simulink model "afsMatrixBeam"  (R2019b)
settings: Solver=FixedStepDiscrete  StartTime=0.0  StopTime=inf  RelTol=1e-3  EnableMultiTasking=on
libraries: SCANeR_API x3
settings Model: Creator=davendano  LastModifiedBy=lpfeffer
settings DataIOCC: LimitDataPoints=on  SaveFormat=Array  ReturnWorkspaceOutputs=off
settings OptimizationCC: LifeSpan=inf
settings DebuggingCC: UnderspecifiedInitializationDetection=Classic  MergeDetectMultiDrivingBlocksExec=none  SolverPrmCheckMsg=warning  SFUnexpectedBacktrackingDiag=warning  SFNoUnconditionalDefaultTransitionDiag=warning  SFExecutionAtInitializationDiag=none  ArithmeticOperatorsInVariantConditions=warning
settings HardwareCC: ProdBitPerPointer=32  ProdBitPerSizeT=32  ProdBitPerPtrDiffT=32  ProdLargestAtomicFloat=None  ProdIntDivRoundTo=Undefined  ProdEndianess=Unspecified  ProdWordSize=32  ProdHWDeviceType=32-bit Generic
settings ModelReferenceCC: PropagateSignalLabelsOutOfModel=off
settings SFSimCC: SimUseLocalCustomCode=off  CustomCodeUndefinedFunction=UseInterfaceOnly
settings RTWCC: Description=OKTAL AFS SCANeR Real-Time Target  SystemTargetFile=grt_CallasPlugin.tlc  TemplateMakefile=grt_moduleOktal  RTWUseLocalCustomCode=off
settings CodeAppCC: StateflowObjectComments=on
settings STFCustomTargetCC: ModelReferenceCompliant=off  GeneratePreprocessorConditionals=Disable all  CombineOutputUpdateFcns=on  MatFileLogging=on  CPPClassGenCompliant=on  SystemTargetFile=grt_CallasPlugin.tlc
settings GRTTargetCC: TargetLangStandard=C89/C90 (ANSI)  ModelReferenceCompliant=off  ParMdlRefBuildCompliant=off  CompOptLevelCompliant=off  ConcurrentExecutionCompliant=off  GeneratePreprocessorConditionals=Disable all  UseToolchainInfoCompliant=off
settings ConfigComp: CovMetricSettings=dw  CovHtmlReporting=on  CovSaveCumulativeToWorkspaceVar=on  CovSaveSingleToWorkspaceVar=on  CovExternalEMLEnable=off

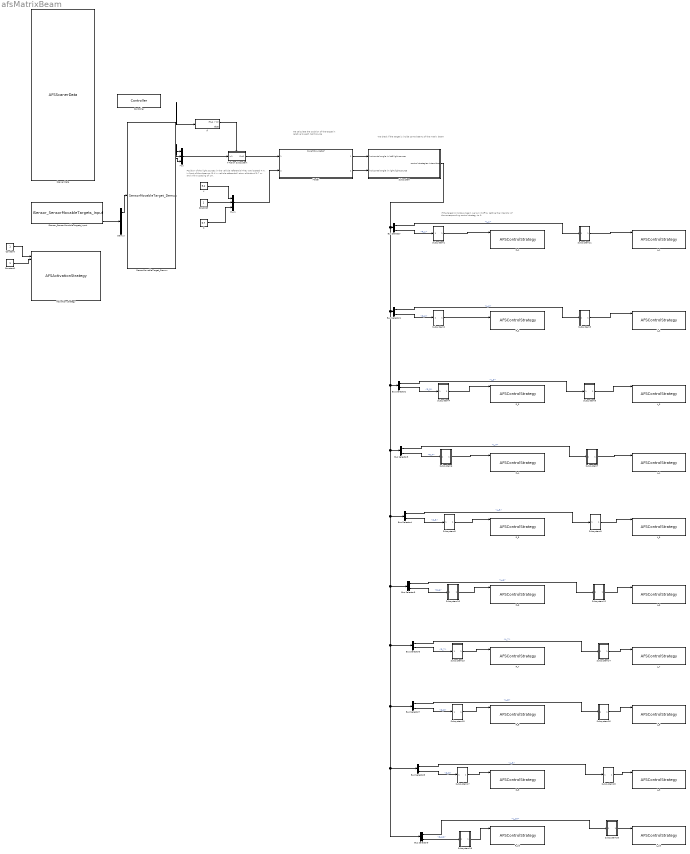
== system afsMatrixBeam ==
  note: If the target is inside a beam we turn it off
      | by setting the intensity of the corresponding control strategy to 0.
  note: We check if the target is inside some beams of the matrix beam
  note: We calculate the position of the target in
      | relative to each light source
  note: Position of the light sources in the vehicle referential
      | They are located 4 m. in front of the observer (5.4 in vehicle referential)
      | at an altitude of 0.7 m. and with a spacing of 1m.
  Activation strategy : S-Function  InitFcn=try, set_param(gcb,'FunctionName','AFSActivationStrategy'), end  FunctionName=AFSActivationStrategy  SFunctionDeploymentMode=off  EnableBusSupport=off  mask(S-Function Builder){}
      mask init:
      | val = [[.9  0.75 0.75 1 1 .9 .9 1]',[1 1 0.75 0.75 .9 .9 1 .9]'];try , sys = get_param(gcb,'SfunBuilderFcnName');if isempty(sys), sys = get_param(gcb,'FunctionName'); end,catch, sys = get_param(gcb,'FunctionName'); end
      settings: CopyFcn=set_param(gcbh,'LinkStatus','none')  PreSaveFcn=try, set_param(gcb,'FunctionName','AFSActivationStrategy'), end
      mask Display:
      | port_label('input',1,'LowBeam')
      | port_label('input',2,'HighBeam')
      | port_label('input',3,'MotorWay')
      | port_label('input',4,'Town')
      | port_label('input',5,'Traffic')
      | port_label('input',6,'AdverseWeather')
      | port_label('input',7,'TurnIndicator')
      | port_label('input',8,'DayTimeRunningLight')
      | port_label('input',9,'ProgressiveBendingLight')
      | port_label('input',10,'CustomBeam1')
      | port_label('input',11,'CustomBeam2')
      | port_label('input',12,'CustomBeam3')
      | fprintf('ACTIVATION\n STRATEGY\n')
  Bus Selector : BusSelector  OutputSignals=L.L_1,R.R_1
  Bus Selector1 : BusSelector  OutputSignals=L.L_2,R.R_2
  Bus Selector2 : BusSelector  OutputSignals=L.L_3,R.R_3
  Bus Selector3 : BusSelector  OutputSignals=L.L_4,R.R_4
  Bus Selector4 : BusSelector  OutputSignals=L.L_5,R.R_5
  Bus Selector5 : BusSelector  OutputSignals=L.L_6,R.R_6
  Bus Selector6 : BusSelector  OutputSignals=L.L_7,R.R_7
  Bus Selector7 : BusSelector  OutputSignals=L.L_8,R.R_8
  Bus Selector8 : BusSelector  OutputSignals=L.L_9,R.R_9
  Bus Selector9 : BusSelector  OutputSignals=L.L_10,R.R_10
  Constant : Constant
  Constant1 : Constant
  Controller : SCANeR_API/Controller  Priority=1  Config='SAMPLE_2022_HEADLIGHTS'  ProcName='SIMULINK'  Frequency=100  NetworkOutputFrequency=10  TimeOut=30  IsSynchronized=off
      settings: SourceProductName=SCANeR API
  Demux : Demux  Outputs=[41 41 41 10373]
  ISensor_SensorMovableTargets_Input : SCANeR_API/Network inputs/ISensor/ISensor_SensorMovableTargets_Input  Priority=2  ev=off  globalId=100000
      settings: SourceProductName=SCANeR API
  If : If
  If Action Subsystem : Subsystem  TreatAsAtomicUnit=on
  L_1 : S-Function  InitFcn=try, set_param(gcb,'FunctionName','AFSControlStrategy'), end  FunctionName=AFSControlStrategy  SFunctionDeploymentMode=off  EnableBusSupport=off  mask(S-Function Builder){}
      mask init: same as afsMatrixBeam/Activation strategy
      settings: CopyFcn=set_param(gcbh,'LinkStatus','none')  PreSaveFcn=try, set_param(gcb,'FunctionName','AFSControlStrategy'), end
      mask Display:
      | port_label('input',1,'Intensity')
      | port_label('input',2,'Heading')
      | port_label('input',3,'Pitch')
      | port_label('input',4,'Roll')
      | fprintf('CONTROL\n STRATEGY\n name:%s\n',get_param(gcb, 'Name'))
  L_10 : S-Function  InitFcn=try, set_param(gcb,'FunctionName','AFSControlStrategy'), end  FunctionName=AFSControlStrategy  SFunctionDeploymentMode=off  EnableBusSupport=off  mask(S-Function Builder){}
      mask init: same as afsMatrixBeam/Activation strategy
      settings: CopyFcn=set_param(gcbh,'LinkStatus','none')  PreSaveFcn=try, set_param(gcb,'FunctionName','AFSControlStrategy'), end
      mask Display:
      | port_label('input',1,'Intensity')
      | port_label('input',2,'Heading')
      | port_label('input',3,'Pitch')
      | port_label('input',4,'Roll')
      | fprintf('CONTROL\n STRATEGY\n name:%s\n',get_param(gcb, 'Name'))
  L_2 : S-Function  InitFcn=try, set_param(gcb,'FunctionName','AFSControlStrategy'), end  FunctionName=AFSControlStrategy  SFunctionDeploymentMode=off  EnableBusSupport=off  mask(S-Function Builder){}
      mask init: same as afsMatrixBeam/Activation strategy
      settings: CopyFcn=set_param(gcbh,'LinkStatus','none')  PreSaveFcn=try, set_param(gcb,'FunctionName','AFSControlStrategy'), end
      mask Display:
      | port_label('input',1,'Intensity')
      | port_label('input',2,'Heading')
      | port_label('input',3,'Pitch')
      | port_label('input',4,'Roll')
      | fprintf('CONTROL\n STRATEGY\n name:%s\n',get_param(gcb, 'Name'))
  L_3 : S-Function  InitFcn=try, set_param(gcb,'FunctionName','AFSControlStrategy'), end  FunctionName=AFSControlStrategy  SFunctionDeploymentMode=off  EnableBusSupport=off  mask(S-Function Builder){}
      mask init: same as afsMatrixBeam/Activation strategy
      settings: CopyFcn=set_param(gcbh,'LinkStatus','none')  PreSaveFcn=try, set_param(gcb,'FunctionName','AFSControlStrategy'), end
      mask Display:
      | port_label('input',1,'Intensity')
      | port_label('input',2,'Heading')
      | port_label('input',3,'Pitch')
      | port_label('input',4,'Roll')
      | fprintf('CONTROL\n STRATEGY\n name:%s\n',get_param(gcb, 'Name'))
  L_4 : S-Function  InitFcn=try, set_param(gcb,'FunctionName','AFSControlStrategy'), end  FunctionName=AFSControlStrategy  SFunctionDeploymentMode=off  EnableBusSupport=off  mask(S-Function Builder){}
      mask init: same as afsMatrixBeam/Activation strategy
      settings: CopyFcn=set_param(gcbh,'LinkStatus','none')  PreSaveFcn=try, set_param(gcb,'FunctionName','AFSControlStrategy'), end
      mask Display:
      | port_label('input',1,'Intensity')
      | port_label('input',2,'Heading')
      | port_label('input',3,'Pitch')
      | port_label('input',4,'Roll')
      | fprintf('CONTROL\n STRATEGY\n name:%s\n',get_param(gcb, 'Name'))
  L_5 : S-Function  InitFcn=try, set_param(gcb,'FunctionName','AFSControlStrategy'), end  FunctionName=AFSControlStrategy  SFunctionDeploymentMode=off  EnableBusSupport=off  mask(S-Function Builder){}
      mask init: same as afsMatrixBeam/Activation strategy
      settings: CopyFcn=set_param(gcbh,'LinkStatus','none')  PreSaveFcn=try, set_param(gcb,'FunctionName','AFSControlStrategy'), end
      mask Display:
      | port_label('input',1,'Intensity')
      | port_label('input',2,'Heading')
      | port_label('input',3,'Pitch')
      | port_label('input',4,'Roll')
      | fprintf('CONTROL\n STRATEGY\n name:%s\n',get_param(gcb, 'Name'))
  L_6 : S-Function  InitFcn=try, set_param(gcb,'FunctionName','AFSControlStrategy'), end  FunctionName=AFSControlStrategy  SFunctionDeploymentMode=off  EnableBusSupport=off  mask(S-Function Builder){}
      mask init: same as afsMatrixBeam/Activation strategy
      settings: CopyFcn=set_param(gcbh,'LinkStatus','none')  PreSaveFcn=try, set_param(gcb,'FunctionName','AFSControlStrategy'), end
      mask Display:
      | port_label('input',1,'Intensity')
      | port_label('input',2,'Heading')
      | port_label('input',3,'Pitch')
      | port_label('input',4,'Roll')
      | fprintf('CONTROL\n STRATEGY\n name:%s\n',get_param(gcb, 'Name'))
  L_7 : S-Function  InitFcn=try, set_param(gcb,'FunctionName','AFSControlStrategy'), end  FunctionName=AFSControlStrategy  SFunctionDeploymentMode=off  EnableBusSupport=off  mask(S-Function Builder){}
      mask init: same as afsMatrixBeam/Activation strategy
      settings: CopyFcn=set_param(gcbh,'LinkStatus','none')  PreSaveFcn=try, set_param(gcb,'FunctionName','AFSControlStrategy'), end
      mask Display:
      | port_label('input',1,'Intensity')
      | port_label('input',2,'Heading')
      | port_label('input',3,'Pitch')
      | port_label('input',4,'Roll')
      | fprintf('CONTROL\n STRATEGY\n name:%s\n',get_param(gcb, 'Name'))
  L_8 : S-Function  InitFcn=try, set_param(gcb,'FunctionName','AFSControlStrategy'), end  FunctionName=AFSControlStrategy  SFunctionDeploymentMode=off  EnableBusSupport=off  mask(S-Function Builder){}
      mask init: same as afsMatrixBeam/Activation strategy
      settings: CopyFcn=set_param(gcbh,'LinkStatus','none')  PreSaveFcn=try, set_param(gcb,'FunctionName','AFSControlStrategy'), end
      mask Display:
      | port_label('input',1,'Intensity')
      | port_label('input',2,'Heading')
      | port_label('input',3,'Pitch')
      | port_label('input',4,'Roll')
      | fprintf('CONTROL\n STRATEGY\n name:%s\n',get_param(gcb, 'Name'))
  L_9 : S-Function  InitFcn=try, set_param(gcb,'FunctionName','AFSControlStrategy'), end  FunctionName=AFSControlStrategy  SFunctionDeploymentMode=off  EnableBusSupport=off  mask(S-Function Builder){}
      mask init: same as afsMatrixBeam/Activation strategy
      settings: CopyFcn=set_param(gcbh,'LinkStatus','none')  PreSaveFcn=try, set_param(gcb,'FunctionName','AFSControlStrategy'), end
      mask Display:
      | port_label('input',1,'Intensity')
      | port_label('input',2,'Heading')
      | port_label('input',3,'Pitch')
      | port_label('input',4,'Roll')
      | fprintf('CONTROL\n STRATEGY\n name:%s\n',get_param(gcb, 'Name'))
  Model : ModelReference  ModelNameDialog=toLightSourceRef.slx  SimulationMode=Normal  ModelReferenceVersion=1.14
  Mux : Mux  Inputs=3
  Mux1 : Mux  Inputs=3
  R_1 : S-Function  InitFcn=try, set_param(gcb,'FunctionName','AFSControlStrategy'), end  FunctionName=AFSControlStrategy  SFunctionDeploymentMode=off  EnableBusSupport=off  mask(S-Function Builder){}
      mask init: same as afsMatrixBeam/Activation strategy
      settings: CopyFcn=set_param(gcbh,'LinkStatus','none')  PreSaveFcn=try, set_param(gcb,'FunctionName','AFSControlStrategy'), end
      mask Display:
      | port_label('input',1,'Intensity')
      | port_label('input',2,'Heading')
      | port_label('input',3,'Pitch')
      | port_label('input',4,'Roll')
      | fprintf('CONTROL\n STRATEGY\n name:%s\n',get_param(gcb, 'Name'))
  R_10 : S-Function  InitFcn=try, set_param(gcb,'FunctionName','AFSControlStrategy'), end  FunctionName=AFSControlStrategy  SFunctionDeploymentMode=off  EnableBusSupport=off  mask(S-Function Builder){}
      mask init: same as afsMatrixBeam/Activation strategy
      settings: CopyFcn=set_param(gcbh,'LinkStatus','none')  PreSaveFcn=try, set_param(gcb,'FunctionName','AFSControlStrategy'), end
      mask Display:
      | port_label('input',1,'Intensity')
      | port_label('input',2,'Heading')
      | port_label('input',3,'Pitch')
      | port_label('input',4,'Roll')
      | fprintf('CONTROL\n STRATEGY\n name:%s\n',get_param(gcb, 'Name'))
  R_2 : S-Function  InitFcn=try, set_param(gcb,'FunctionName','AFSControlStrategy'), end  FunctionName=AFSControlStrategy  SFunctionDeploymentMode=off  EnableBusSupport=off  mask(S-Function Builder){}
      mask init: same as afsMatrixBeam/Activation strategy
      settings: CopyFcn=set_param(gcbh,'LinkStatus','none')  PreSaveFcn=try, set_param(gcb,'FunctionName','AFSControlStrategy'), end
      mask Display:
      | port_label('input',1,'Intensity')
      | port_label('input',2,'Heading')
      | port_label('input',3,'Pitch')
      | port_label('input',4,'Roll')
      | fprintf('CONTROL\n STRATEGY\n name:%s\n',get_param(gcb, 'Name'))
  R_3 : S-Function  InitFcn=try, set_param(gcb,'FunctionName','AFSControlStrategy'), end  FunctionName=AFSControlStrategy  SFunctionDeploymentMode=off  EnableBusSupport=off  mask(S-Function Builder){}
      mask init: same as afsMatrixBeam/Activation strategy
      settings: CopyFcn=set_param(gcbh,'LinkStatus','none')  PreSaveFcn=try, set_param(gcb,'FunctionName','AFSControlStrategy'), end
      mask Display:
      | port_label('input',1,'Intensity')
      | port_label('input',2,'Heading')
      | port_label('input',3,'Pitch')
      | port_label('input',4,'Roll')
      | fprintf('CONTROL\n STRATEGY\n name:%s\n',get_param(gcb, 'Name'))
  R_4 : S-Function  InitFcn=try, set_param(gcb,'FunctionName','AFSControlStrategy'), end  FunctionName=AFSControlStrategy  SFunctionDeploymentMode=off  EnableBusSupport=off  mask(S-Function Builder){}
      mask init: same as afsMatrixBeam/Activation strategy
      settings: CopyFcn=set_param(gcbh,'LinkStatus','none')  PreSaveFcn=try, set_param(gcb,'FunctionName','AFSControlStrategy'), end
      mask Display:
      | port_label('input',1,'Intensity')
      | port_label('input',2,'Heading')
      | port_label('input',3,'Pitch')
      | port_label('input',4,'Roll')
      | fprintf('CONTROL\n STRATEGY\n name:%s\n',get_param(gcb, 'Name'))
  R_5 : S-Function  InitFcn=try, set_param(gcb,'FunctionName','AFSControlStrategy'), end  FunctionName=AFSControlStrategy  SFunctionDeploymentMode=off  EnableBusSupport=off  mask(S-Function Builder){}
      mask init: same as afsMatrixBeam/Activation strategy
      settings: CopyFcn=set_param(gcbh,'LinkStatus','none')  PreSaveFcn=try, set_param(gcb,'FunctionName','AFSControlStrategy'), end
      mask Display:
      | port_label('input',1,'Intensity')
      | port_label('input',2,'Heading')
      | port_label('input',3,'Pitch')
      | port_label('input',4,'Roll')
      | fprintf('CONTROL\n STRATEGY\n name:%s\n',get_param(gcb, 'Name'))
  R_6 : S-Function  InitFcn=try, set_param(gcb,'FunctionName','AFSControlStrategy'), end  FunctionName=AFSControlStrategy  SFunctionDeploymentMode=off  EnableBusSupport=off  mask(S-Function Builder){}
      mask init: same as afsMatrixBeam/Activation strategy
      settings: CopyFcn=set_param(gcbh,'LinkStatus','none')  PreSaveFcn=try, set_param(gcb,'FunctionName','AFSControlStrategy'), end
      mask Display:
      | port_label('input',1,'Intensity')
      | port_label('input',2,'Heading')
      | port_label('input',3,'Pitch')
      | port_label('input',4,'Roll')
      | fprintf('CONTROL\n STRATEGY\n name:%s\n',get_param(gcb, 'Name'))
  R_7 : S-Function  InitFcn=try, set_param(gcb,'FunctionName','AFSControlStrategy'), end  FunctionName=AFSControlStrategy  SFunctionDeploymentMode=off  EnableBusSupport=off  mask(S-Function Builder){}
      mask init: same as afsMatrixBeam/Activation strategy
      settings: CopyFcn=set_param(gcbh,'LinkStatus','none')  PreSaveFcn=try, set_param(gcb,'FunctionName','AFSControlStrategy'), end
      mask Display:
      | port_label('input',1,'Intensity')
      | port_label('input',2,'Heading')
      | port_label('input',3,'Pitch')
      | port_label('input',4,'Roll')
      | fprintf('CONTROL\n STRATEGY\n name:%s\n',get_param(gcb, 'Name'))
  R_8 : S-Function  InitFcn=try, set_param(gcb,'FunctionName','AFSControlStrategy'), end  FunctionName=AFSControlStrategy  SFunctionDeploymentMode=off  EnableBusSupport=off  mask(S-Function Builder){}
      mask init: same as afsMatrixBeam/Activation strategy
      settings: CopyFcn=set_param(gcbh,'LinkStatus','none')  PreSaveFcn=try, set_param(gcb,'FunctionName','AFSControlStrategy'), end
      mask Display:
      | port_label('input',1,'Intensity')
      | port_label('input',2,'Heading')
      | port_label('input',3,'Pitch')
      | port_label('input',4,'Roll')
      | fprintf('CONTROL\n STRATEGY\n name:%s\n',get_param(gcb, 'Name'))
  R_9 : S-Function  InitFcn=try, set_param(gcb,'FunctionName','AFSControlStrategy'), end  FunctionName=AFSControlStrategy  SFunctionDeploymentMode=off  EnableBusSupport=off  mask(S-Function Builder){}
      mask init: same as afsMatrixBeam/Activation strategy
      settings: CopyFcn=set_param(gcbh,'LinkStatus','none')  PreSaveFcn=try, set_param(gcb,'FunctionName','AFSControlStrategy'), end
      mask Display:
      | port_label('input',1,'Intensity')
      | port_label('input',2,'Heading')
      | port_label('input',3,'Pitch')
      | port_label('input',4,'Roll')
      | fprintf('CONTROL\n STRATEGY\n name:%s\n',get_param(gcb, 'Name'))
  SPACING : Constant
  Scaner Data : S-Function  InitFcn=try, set_param(gcb,'FunctionName','AFSScanerData'), end  FunctionName=AFSScanerData  Parameters=Frequency  SFunctionDeploymentMode=off  EnableBusSupport=off  mask(S-Function Builder){Frequency=100}
      mask prompts: Frequency "Frequency (Hz) (use 0 when used with SCANeR API)"
      mask init: same as afsMatrixBeam/Activation strategy
      settings: CopyFcn=set_param(gcbh,'LinkStatus','none')  PreSaveFcn=try, set_param(gcb,'FunctionName','AFSScanerData'), end
      mask Display:
      | port_label('output',1,'Speed')
      | port_label('output',2,'SteeringWheelAngle')
      | port_label('output',3,'CurrentCurveCurvature')
      | port_label('output',4,'CurveCurvatureAtXMeters')
      | port_label('output',5,'TheoreticalTime')
      | port_label('output',6,'MeasuredTime')
      | port_label('output',7,'X')
      | port_label('output',8,'Y')
      | port_label('output',9,'Z')
      | port_label('output',10,'Heading')
      | port_label('output',11,'Pitch')
      | port_label('output',12,'Roll')
      | port_label('output',13,'HeadingRelativeToTheRoad')
      | port_label('output',14,'GeographicClassification')
      | port_label('output',15,'GearBox')
      | port_label('output',16,'Indicators')
      | port_label('output',17,'Warning')
      | port_label('output',18,'LightStatus')
      | port_label('output',19,'LongitudinalAcceleration')
      | port_label('output',20,'DistanceToNextVehicleInSameDirection')
      | port_label('output',21,'DistanceToNextVehicleInOppositeDirection')
      | port_label('output',22,'SnowLevel')
      | port_label('output',23,'RainLevel')
      | port_label('output',24,'FogDistance')
      | port_label('output',25,'BrakePedal')
      | port_label('output',26,'AcceleratorPedal')
      | port_label('output',27,'VehicleLoad')
      | port_label('output',28,'RemoteHeightAdjustmentHeadlamp')
      | port_label('output',29,'SteerAngle')
      | port_label('output',30,'Wheelbase')
      | port_label('output',31,'AngularVelocityHeading')
      | port_label('output',32,'Traffic')
      | port_label('output',33,'CustomInput')
      | port_label('output',34,'CustomOutput')
      | fprintf('SCANeR\n DATA\n')
  SensorMovableTarget_Demux : SCANeR_API/Structures/SensorMovableTarget_Demux
      settings: SourceProductName=SCANeR API
  Subsystem : Subsystem
  Subsystem1 : Subsystem
  Subsystem10 : Subsystem
  Subsystem11 : Subsystem
  Subsystem12 : Subsystem
  Subsystem13 : Subsystem
  Subsystem14 : Subsystem
  Subsystem15 : Subsystem
  Subsystem16 : Subsystem
  Subsystem17 : Subsystem
  Subsystem18 : Subsystem
  Subsystem19 : Subsystem
  Subsystem2 : Subsystem
  Subsystem20 : Subsystem
  Subsystem3 : Subsystem
  Subsystem4 : Subsystem
  Subsystem5 : Subsystem
  Subsystem6 : Subsystem
  Subsystem7 : Subsystem
  Subsystem8 : Subsystem
  Subsystem9 : Subsystem
  X : Constant  Value=5.4
  Z : Constant  Value=0.7
  wires:
  Constant/1 -> Activation strategy/1
  Constant1/1 -> Activation strategy/2
  ISensor_SensorMovableTargets_Input/6 -> Demux/1
  Demux/1 -> SensorMovableTarget_Demux/1
  SensorMovableTarget_Demux/10 -> Mux/2
  SensorMovableTarget_Demux/9 -> Mux/1
  SensorMovableTarget_Demux/11 -> Mux/3
  Mux/1 -> If Action Subsystem/1(In1)
  X/1 -> Mux1/1
  SPACING/1 -> Mux1/2
  Z/1 -> Mux1/3
  Mux1/1 -> Model/2
  Model/1 -> Subsystem/1(horizontal angle in left light source)
  Model/2 -> Subsystem/2(horizontal angle in right light source)
  Subsystem/1(control strategies intensities) -> Bus Selector9/1, Bus Selector8/1, Bus Selector7/1, Bus Selector6/1, Bus Selector5/1, Bus Selector4/1, Bus Selector3/1, Bus Selector2/1, Bus Selector1/1, Bus Selector/1
  Bus Selector/2 -> Subsystem1/1(In1)  "<R_1>"
  Subsystem1/1(Out1) -> R_1/1
  Bus Selector/1 -> Subsystem11/1(In1)  "<L_1>"
  Subsystem11/1(Out1) -> L_1/1
  Bus Selector1/2 -> Subsystem2/1(In1)  "<R_2>"
  Subsystem2/1(Out1) -> R_2/2
  Bus Selector1/1 -> Subsystem3/1(In1)  "<L_2>"
  Subsystem3/1(Out1) -> L_2/1
  Bus Selector2/2 -> Subsystem4/1(In1)  "<R_3>"
  Subsystem4/1(Out1) -> R_3/1
  Bus Selector2/1 -> Subsystem5/1(In1)  "<L_3>"
  Subsystem5/1(Out1) -> L_3/1
  Bus Selector3/2 -> Subsystem6/1(In1)  "<R_4>"
  Subsystem6/1(Out1) -> R_4/1
  Bus Selector3/1 -> Subsystem7/1(In1)  "<L_4>"
  Subsystem7/1(Out1) -> L_4/1
  Bus Selector4/2 -> Subsystem8/1(In1)  "<R_5>"
  Subsystem8/1(Out1) -> R_5/1
  Bus Selector4/1 -> Subsystem9/1(In1)  "<L_5>"
  Subsystem9/1(Out1) -> L_5/1
  Bus Selector5/2 -> Subsystem10/1(In1)  "<R_6>"
  Subsystem10/1(Out1) -> R_6/1
  Bus Selector5/1 -> Subsystem12/1(In1)  "<L_6>"
  Subsystem12/1(Out1) -> L_6/1
  Bus Selector6/2 -> Subsystem13/1(In1)  "<R_7>"
  Subsystem13/1(Out1) -> R_7/1
  Bus Selector6/1 -> Subsystem14/1(In1)  "<L_7>"
  Subsystem14/1(Out1) -> L_7/1
  Bus Selector7/2 -> Subsystem15/1(In1)  "<R_8>"
  Subsystem15/1(Out1) -> R_8/1
  Bus Selector7/1 -> Subsystem16/1(In1)  "<L_8>"
  Subsystem16/1(Out1) -> L_8/1
  Bus Selector8/2 -> Subsystem17/1(In1)  "<R_9>"
  Subsystem17/1(Out1) -> R_9/1
  Bus Selector8/1 -> Subsystem18/1(In1)  "<L_9>"
  Subsystem18/1(Out1) -> L_9/1
  Bus Selector9/2 -> Subsystem19/1(In1)  "<R_10>"
  Subsystem19/1(Out1) -> R_10/1
  Bus Selector9/1 -> Subsystem20/1(In1)  "<L_10>"
  Subsystem20/1(Out1) -> L_10/1
  SensorMovableTarget_Demux/1 -> If/1
  If Action Subsystem/1(Out1) -> Model/1
  If/1 -> If Action Subsystem/Action

== system afsMatrixBeam/If Action Subsystem ==
  In1 : Inport
  Action Port : ActionPort  ActionPortLabel=if { }
  Out1 : Outport
  wires:
  In1/1 -> Out1/1

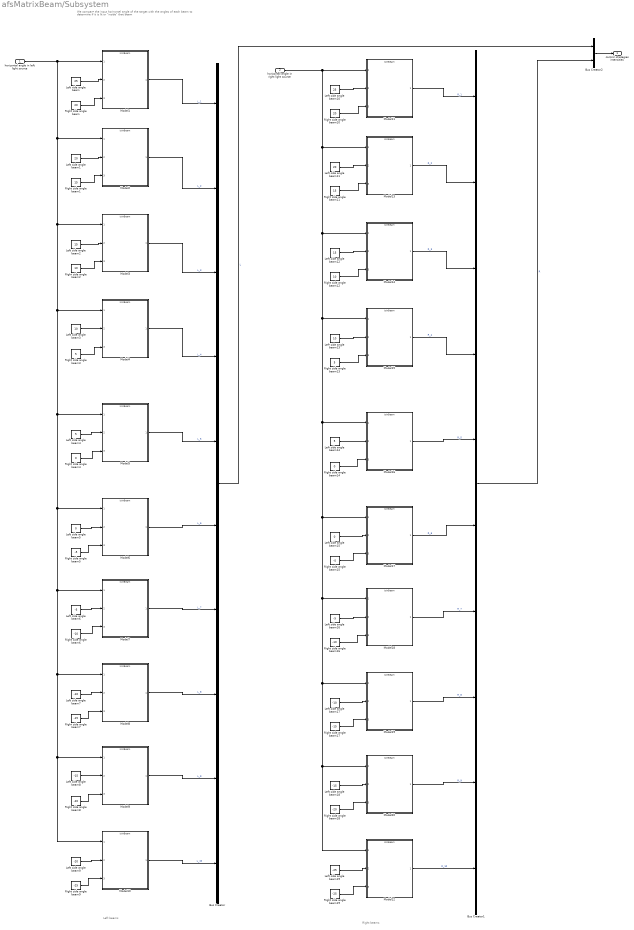
== system afsMatrixBeam/Subsystem ==
  note: Right beams
  note: Left beams
  note: We compare the input horizontal angle of the target with the angles of each beam
      | to determine if it is lit or "inside" that beam
  horizontal angle in left light source : Inport
  horizontal angle in right light source : Inport  Port=2
  Bus Creator : BusCreator  Inputs=10
  Bus Creator1 : BusCreator  Inputs=10
  Bus Creator2 : BusCreator  Inputs=2
  Left side angle beam : Constant  Value=25
  Left side angle beam1 : Constant  Value=20
  Left side angle beam10 : Constant  Value=25
  Left side angle beam11 : Constant  Value=20
  Left side angle beam12 : Constant  Value=15
  Left side angle beam13 : Constant  Value=10
  Left side angle beam14 : Constant  Value=5
  Left side angle beam15 : Constant  Value=0
  Left side angle beam16 : Constant  Value=-5
  Left side angle beam17 : Constant  Value=-10
  Left side angle beam18 : Constant  Value=-15
  Left side angle beam19 : Constant  Value=-25
  Left side angle beam2 : Constant  Value=15
  Left side angle beam3 : Constant  Value=10
  Left side angle beam4 : Constant  Value=5
  Left side angle beam5 : Constant  Value=0
  Left side angle beam6 : Constant  Value=-5
  Left side angle beam7 : Constant  Value=-10
  Left side angle beam8 : Constant  Value=-15
  Left side angle beam9 : Constant  Value=-20
  Model{1..20} (20 alike) : ModelReference  ModelNameDialog=isInBeam.slx  SimulationMode=Normal  ModelReferenceVersion=1.7
  Right side angle beam : Constant  Value=20
  Right side angle beam1 : Constant  Value=15
  Right side angle beam10 : Constant  Value=20
  Right side angle beam11 : Constant  Value=15
  Right side angle beam12 : Constant  Value=10
  Right side angle beam13 : Constant  Value=5
  Right side angle beam14 : Constant  Value=0
  Right side angle beam15 : Constant  Value=-5
  Right side angle beam16 : Constant  Value=-10
  Right side angle beam17 : Constant  Value=-15
  Right side angle beam18 : Constant  Value=-20
  Right side angle beam19 : Constant  Value=-25
  Right side angle beam2 : Constant  Value=10
  Right side angle beam3 : Constant  Value=5
  Right side angle beam4 : Constant  Value=0
  Right side angle beam5 : Constant  Value=-5
  Right side angle beam6 : Constant  Value=-10
  Right side angle beam7 : Constant  Value=-15
  Right side angle beam8 : Constant  Value=-20
  Right side angle beam9 : Constant  Value=-25
  control strategies intensities : Outport
  wires:
  Left side angle beam4/1 -> Model5/2
  Right side angle beam4/1 -> Model5/3
  Right side angle beam1/1 -> Model2/3
  Left side angle beam1/1 -> Model2/2
  Left side angle beam7/1 -> Model8/2
  Right side angle beam7/1 -> Model8/3
  Left side angle beam2/1 -> Model3/2
  Right side angle beam2/1 -> Model3/3
  Left side angle beam5/1 -> Model6/2
  Right side angle beam5/1 -> Model6/3
  Model6/1 -> Bus Creator/6  "L_6"
  Left side angle beam9/1 -> Model10/2
  horizontal angle in left light source/1 -> Model10/1, Model9/1, Model8/1, Model7/1, Model6/1, Model5/1, Model4/1, Model3/1, Model2/1, Model1/1
  Model10/1 -> Bus Creator/10  "L_10"
  Right side angle beam9/1 -> Model10/3
  Model4/1 -> Bus Creator/4  "L_4"
  Model9/1 -> Bus Creator/9  "L_9"
  Model7/1 -> Bus Creator/7  "L_7"
  Model1/1 -> Bus Creator/1  "L_1"
  Model2/1 -> Bus Creator/2  "L_2"
  Model5/1 -> Bus Creator/5  "L_5"
  Model3/1 -> Bus Creator/3  "L_3"
  Model8/1 -> Bus Creator/8  "L_8"
  Right side angle beam3/1 -> Model4/3
  Left side angle beam3/1 -> Model4/2
  Right side angle beam8/1 -> Model9/3
  Left side angle beam8/1 -> Model9/2
  Right side angle beam/1 -> Model1/3
  Left side angle beam/1 -> Model1/2
  Left side angle beam6/1 -> Model7/2
  Right side angle beam6/1 -> Model7/3
  Left side angle beam14/1 -> Model16/2
  Right side angle beam14/1 -> Model16/3
  Right side angle beam11/1 -> Model13/3
  Left side angle beam11/1 -> Model13/2
  Left side angle beam17/1 -> Model19/2
  Right side angle beam17/1 -> Model19/3
  Left side angle beam12/1 -> Model14/2
  Right side angle beam12/1 -> Model14/3
  Left side angle beam15/1 -> Model17/2
  Right side angle beam15/1 -> Model17/3
  Model17/1 -> Bus Creator1/6  "R_6"
  Left side angle beam19/1 -> Model12/2
  horizontal angle in right light source/1 -> Model11/1, Model13/1, Model14/1, Model15/1, Model16/1, Model17/1, Model18/1, Model19/1, Model20/1, Model12/1
  Model12/1 -> Bus Creator1/10  "R_10"
  Right side angle beam19/1 -> Model12/3
  Model15/1 -> Bus Creator1/4  "R_4"
  Model20/1 -> Bus Creator1/9  "R_9"
  Model18/1 -> Bus Creator1/7  "R_7"
  Model11/1 -> Bus Creator1/1  "R_1"
  Model13/1 -> Bus Creator1/2  "R_2"
  Model16/1 -> Bus Creator1/5  "R_5"
  Model14/1 -> Bus Creator1/3  "R_3"
  Model19/1 -> Bus Creator1/8  "R_8"
  Right side angle beam13/1 -> Model15/3
  Left side angle beam13/1 -> Model15/2
  Right side angle beam18/1 -> Model20/3
  Left side angle beam18/1 -> Model20/2
  Right side angle beam10/1 -> Model11/3
  Left side angle beam10/1 -> Model11/2
  Left side angle beam16/1 -> Model18/2
  Right side angle beam16/1 -> Model18/3
  Bus Creator/1 -> Bus Creator2/1  "L"
  Bus Creator1/1 -> Bus Creator2/2  "R"
  Bus Creator2/1 -> control strategies intensities/1

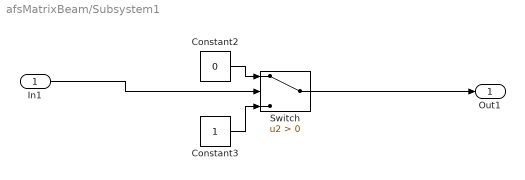
== system afsMatrixBeam/Subsystem1 ==
  In1 : Inport
  Constant2 : Constant  Value=0
  Constant3 : Constant
  Switch : Switch  Criteria=u2 > Threshold
  Out1 : Outport
  wires:
  Constant2/1 -> Switch/1
  Constant3/1 -> Switch/3
  In1/1 -> Switch/2
  Switch/1 -> Out1/1

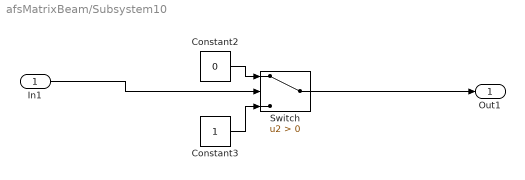
== system afsMatrixBeam/Subsystem10 ==
  In1 : Inport
  Constant2 : Constant  Value=0
  Constant3 : Constant
  Switch : Switch  Criteria=u2 > Threshold
  Out1 : Outport
  wires:
  Switch/1 -> Out1/1
  In1/1 -> Switch/2
  Constant3/1 -> Switch/3
  Constant2/1 -> Switch/1

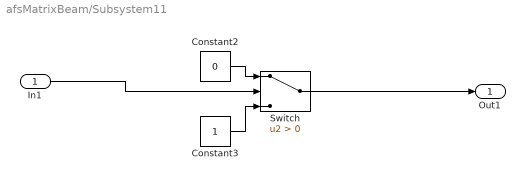
== system afsMatrixBeam/Subsystem11 ==
  In1 : Inport
  Constant2 : Constant  Value=0
  Constant3 : Constant
  Switch : Switch  Criteria=u2 > Threshold
  Out1 : Outport
  wires:
  Switch/1 -> Out1/1
  In1/1 -> Switch/2
  Constant3/1 -> Switch/3
  Constant2/1 -> Switch/1

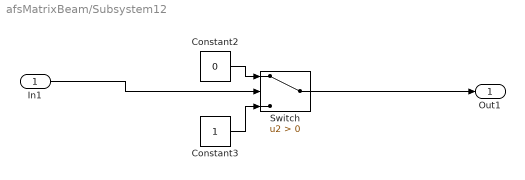
== system afsMatrixBeam/Subsystem12 ==
  In1 : Inport
  Constant2 : Constant  Value=0
  Constant3 : Constant
  Switch : Switch  Criteria=u2 > Threshold
  Out1 : Outport
  wires:
  Constant2/1 -> Switch/1
  Constant3/1 -> Switch/3
  In1/1 -> Switch/2
  Switch/1 -> Out1/1

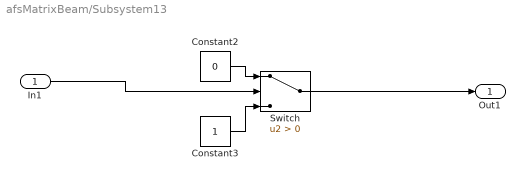
== system afsMatrixBeam/Subsystem13 ==
  In1 : Inport
  Constant2 : Constant  Value=0
  Constant3 : Constant
  Switch : Switch  Criteria=u2 > Threshold
  Out1 : Outport
  wires:
  Constant2/1 -> Switch/1
  Constant3/1 -> Switch/3
  In1/1 -> Switch/2
  Switch/1 -> Out1/1

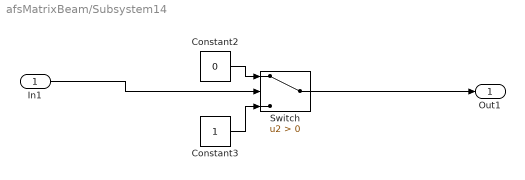
== system afsMatrixBeam/Subsystem14 ==
  In1 : Inport
  Constant2 : Constant  Value=0
  Constant3 : Constant
  Switch : Switch  Criteria=u2 > Threshold
  Out1 : Outport
  wires:
  Switch/1 -> Out1/1
  In1/1 -> Switch/2
  Constant3/1 -> Switch/3
  Constant2/1 -> Switch/1

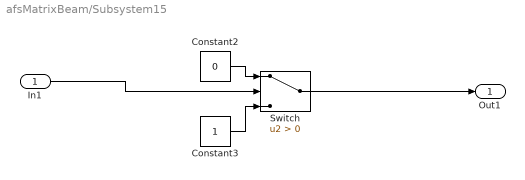
== system afsMatrixBeam/Subsystem15 ==
  In1 : Inport
  Constant2 : Constant  Value=0
  Constant3 : Constant
  Switch : Switch  Criteria=u2 > Threshold
  Out1 : Outport
  wires:
  Switch/1 -> Out1/1
  In1/1 -> Switch/2
  Constant3/1 -> Switch/3
  Constant2/1 -> Switch/1

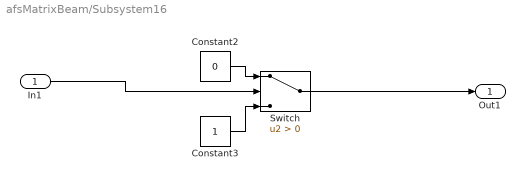
== system afsMatrixBeam/Subsystem16 ==
  In1 : Inport
  Constant2 : Constant  Value=0
  Constant3 : Constant
  Switch : Switch  Criteria=u2 > Threshold
  Out1 : Outport
  wires:
  Constant2/1 -> Switch/1
  Constant3/1 -> Switch/3
  In1/1 -> Switch/2
  Switch/1 -> Out1/1

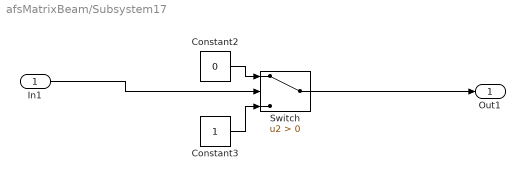
== system afsMatrixBeam/Subsystem17 ==
  In1 : Inport
  Constant2 : Constant  Value=0
  Constant3 : Constant
  Switch : Switch  Criteria=u2 > Threshold
  Out1 : Outport
  wires:
  Constant2/1 -> Switch/1
  Constant3/1 -> Switch/3
  In1/1 -> Switch/2
  Switch/1 -> Out1/1

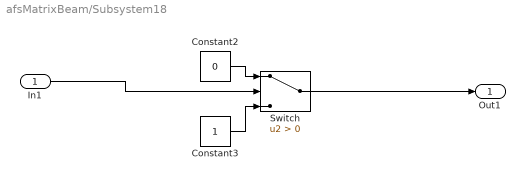
== system afsMatrixBeam/Subsystem18 ==
  In1 : Inport
  Constant2 : Constant  Value=0
  Constant3 : Constant
  Switch : Switch  Criteria=u2 > Threshold
  Out1 : Outport
  wires:
  Switch/1 -> Out1/1
  In1/1 -> Switch/2
  Constant3/1 -> Switch/3
  Constant2/1 -> Switch/1

== system afsMatrixBeam/Subsystem19 ==
  In1 : Inport
  Constant2 : Constant  Value=0
  Constant3 : Constant
  Switch : Switch  Criteria=u2 > Threshold
  Out1 : Outport
  wires:
  Switch/1 -> Out1/1
  In1/1 -> Switch/2
  Constant3/1 -> Switch/3
  Constant2/1 -> Switch/1

== system afsMatrixBeam/Subsystem2 ==
  In1 : Inport
  Constant2 : Constant  Value=0
  Constant3 : Constant
  Switch : Switch  Criteria=u2 > Threshold
  Out1 : Outport
  wires:
  Switch/1 -> Out1/1
  In1/1 -> Switch/2
  Constant3/1 -> Switch/3
  Constant2/1 -> Switch/1

== system afsMatrixBeam/Subsystem20 ==
  In1 : Inport
  Constant2 : Constant  Value=0
  Constant3 : Constant
  Switch : Switch  Criteria=u2 > Threshold
  Out1 : Outport
  wires:
  Constant2/1 -> Switch/1
  Constant3/1 -> Switch/3
  In1/1 -> Switch/2
  Switch/1 -> Out1/1

== system afsMatrixBeam/Subsystem3 ==
  In1 : Inport
  Constant2 : Constant  Value=0
  Constant3 : Constant
  Switch : Switch  Criteria=u2 > Threshold
  Out1 : Outport
  wires:
  Constant2/1 -> Switch/1
  Constant3/1 -> Switch/3
  In1/1 -> Switch/2
  Switch/1 -> Out1/1

== system afsMatrixBeam/Subsystem4 ==
  In1 : Inport
  Constant2 : Constant  Value=0
  Constant3 : Constant
  Switch : Switch  Criteria=u2 > Threshold
  Out1 : Outport
  wires:
  Constant2/1 -> Switch/1
  Constant3/1 -> Switch/3
  In1/1 -> Switch/2
  Switch/1 -> Out1/1

== system afsMatrixBeam/Subsystem5 ==
  In1 : Inport
  Constant2 : Constant  Value=0
  Constant3 : Constant
  Switch : Switch  Criteria=u2 > Threshold
  Out1 : Outport
  wires:
  Switch/1 -> Out1/1
  In1/1 -> Switch/2
  Constant3/1 -> Switch/3
  Constant2/1 -> Switch/1

== system afsMatrixBeam/Subsystem6 ==
  In1 : Inport
  Constant2 : Constant  Value=0
  Constant3 : Constant
  Switch : Switch  Criteria=u2 > Threshold
  Out1 : Outport
  wires:
  Switch/1 -> Out1/1
  In1/1 -> Switch/2
  Constant3/1 -> Switch/3
  Constant2/1 -> Switch/1

== system afsMatrixBeam/Subsystem7 ==
  In1 : Inport
  Constant2 : Constant  Value=0
  Constant3 : Constant
  Switch : Switch  Criteria=u2 > Threshold
  Out1 : Outport
  wires:
  Constant2/1 -> Switch/1
  Constant3/1 -> Switch/3
  In1/1 -> Switch/2
  Switch/1 -> Out1/1

== system afsMatrixBeam/Subsystem8 ==
  In1 : Inport
  Constant2 : Constant  Value=0
  Constant3 : Constant
  Switch : Switch  Criteria=u2 > Threshold
  Out1 : Outport
  wires:
  Constant2/1 -> Switch/1
  Constant3/1 -> Switch/3
  In1/1 -> Switch/2
  Switch/1 -> Out1/1

== system afsMatrixBeam/Subsystem9 ==
  In1 : Inport
  Constant2 : Constant  Value=0
  Constant3 : Constant
  Switch : Switch  Criteria=u2 > Threshold
  Out1 : Outport
  wires:
  Switch/1 -> Out1/1
  In1/1 -> Switch/2
  Constant3/1 -> Switch/3
  Constant2/1 -> Switch/1
